simulink model "pendulum_ADRC_sim_sol"  (R2023b)
settings: Solver=ode3  StartTime=0.0  StopTime=20  FixedStep=0.01  RelTol=1e-3
values from neighbouring files (symbols this model uses):
  A = [ 0 1 ; 0 -a_m ]    [antenna_ADRC_par_sol.m]    (also in antenna_OFB_par_sol.m; pendulum_ADRC_par_sol.m = [ 0 , 1 , 0 ; 0 , 0 , 1 ; 0 , 0 , 0 ])
  a = [ m ; g ; l ; d ]    [pendulum_ADRC_par_sol.m]
  B = [ 0 ; Kl*Kg ]    [antenna_ADRC_par_sol.m]    (also in antenna_OFB_par_sol.m; pendulum_ADRC_par_sol.m = [ 0; b0 ; 0 ])
  b0 = 1/m    (= 0.02)    [pendulum_ADRC_par_sol.m]
  C = [ 1 , 0 ]    [antenna_ADRC_par_sol.m]    (also in antenna_OFB_par_sol.m; pendulum_ADRC_par_sol.m = [ 1 , 0 , 0 ])
  KD = 2*pole_CL    (= 3)    [pendulum_ADRC_par_sol.m]
  KP = pole_CL^2    (= 2.25)    [pendulum_ADRC_par_sol.m]
  L = acker(A',C',p_obs)'    [antenna_OFB_par_sol.m]    (also in pendulum_ADRC_par_sol.m = acker(A',C',poles_ESO)')
libraries: simulink_extras x3
settings Model: Creator=jerome  LastModifiedBy=jerome
settings ModelReferenceCC: EnableRefExpFcnMdlSchedulingChecks=on

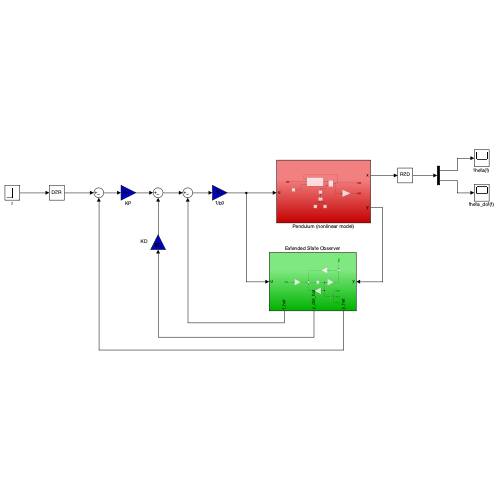
[thumbnail: Simulink's stored preview of the top-level diagram]
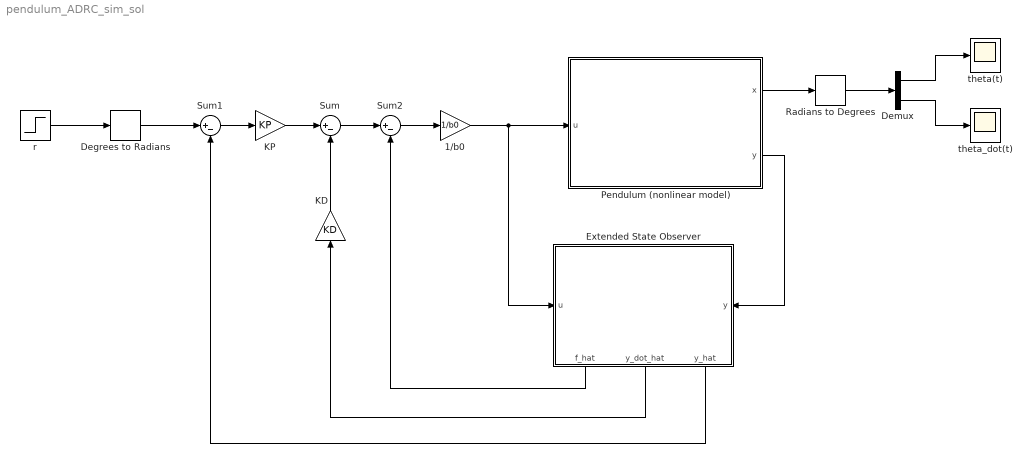
== system pendulum_ADRC_sim_sol ==
  1/b0 : Gain  Gain=1/b0
  Degrees to Radians : simulink_extras/Transformations/Degrees to Radians
  Demux : Demux  Outputs=2
  Extended State Observer : Subsystem
      settings: PortSchema="{\"entries\":[{\"content\":{\"sides\":[{\"content\":{\"connectorIds\":[\"In1\"]},\"type\":\"ConnectorPlacement.EquallySpacedRectSide\",\"uuid\":\"e39c489f-7ce3-4515-bfb3-5978cf16689b\"},{\"content\":{\"connectorIds\":[\"In2\"],\"side\":\"RIGHT\"},\"type\":\"ConnectorPlacement.EquallySpacedRectSide\",\"uuid\":\"c323375b-3042-4327-9d10-0e78d49b9c28\"},{\"content\":{\"connectorIds\":[],\"side\":\"TOP\"},\"type\":\"ConnectorPlacement.EquallySpacedRectSide\",\"uuid\":\"bc6e3c93-589b-408b-8e2a-2332a4933e23\"},{\"content\":{\"connectorIds\":[\"Out1\",\"Out2\",\"Out3\"],\"side\":\"BOTTOM\"},\"type\":\"ConnectorPlacement.EquallySpacedRectSide\",\"uuid\":\"0fa3e6d2-737b-4634-8e4c-4849dc2892cb\"}]},\"type\":\"ConnectorPlacement.EquallySpacedConnector\",\"uuid\":\"052b3b38-b01c-47b0-92b2-1f2c82c768d4\"}],\"packageUris\":[\"http://schema.mathworks.com/mf0/Connector/R2020b\"],\"version\":\"1.0\"}"
  KD : Gain  Gain=KD
  KP : Gain  Gain=KP
  Pendulum (nonlinear model) : Subsystem
  Radians to Degrees : simulink_extras/Transformations/Radians to Degrees
  Sum : Sum  Inputs=|+-
  Sum1 : Sum  Inputs=|+-
  Sum2 : Sum  Inputs=|+-
  r : Step  After=45  SampleTime=0
  theta(t) : Scope
  theta_dot(t) : Scope
  wires:
  KP/1 -> Sum/1
  Sum1/1 -> KP/1
  Extended State Observer/3(y_hat) -> Sum1/2
  Sum2/1 -> 1/b0/1
  Sum/1 -> Sum2/1
  Extended State Observer/1(f_hat) -> Sum2/2
  Extended State Observer/2(y_dot_hat) -> KD/1
  KD/1 -> Sum/2
  Pendulum (nonlinear model)/1(x) -> Radians to Degrees/1
  Radians to Degrees/1 -> Demux/1
  Demux/1 -> theta(t)/1
  Demux/2 -> theta_dot(t)/1
  Pendulum (nonlinear model)/2(y) -> Extended State Observer/2(y)
  1/b0/1 -> Extended State Observer/1(u), Pendulum (nonlinear model)/1(u)
  Degrees to Radians/1 -> Sum1/1
  r/1 -> Degrees to Radians/1

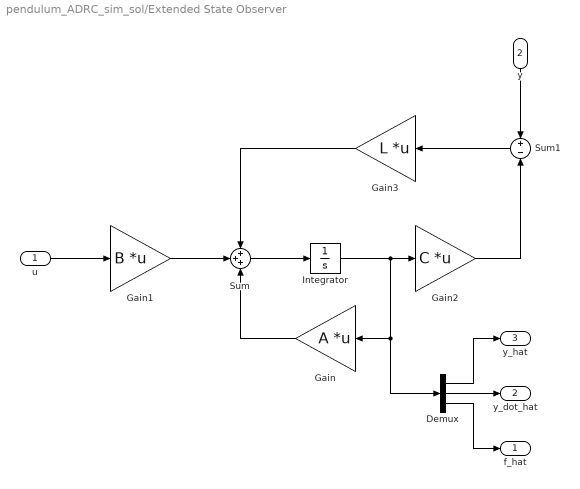
== system pendulum_ADRC_sim_sol/Extended State Observer ==
  u : Inport
  y : Inport  Port=2
  Demux : Demux  Outputs=3
  Gain : Gain  Gain=A  Multiplication=Matrix(K*u) (u vector)
  Gain1 : Gain  Gain=B  Multiplication=Matrix(K*u) (u vector)
  Gain2 : Gain  Gain=C  Multiplication=Matrix(K*u) (u vector)
  Gain3 : Gain  Gain=L  Multiplication=Matrix(K*u) (u vector)
  Integrator : Integrator  InitialCondition=zeros(3,1)
  Sum : Sum  Inputs=+++
  Sum1 : Sum  Inputs=+-
  f_hat : Outport
  y_dot_hat : Outport  Port=2
  y_hat : Outport  Port=3
  wires:
  Integrator/1 -> Gain2/1, Demux/1, Gain/1
  Demux/1 -> y_hat/1
  Sum/1 -> Integrator/1
  u/1 -> Gain1/1
  Gain/1 -> Sum/3
  Gain1/1 -> Sum/2
  Gain3/1 -> Sum/1
  Sum1/1 -> Gain3/1
  Gain2/1 -> Sum1/2
  y/1 -> Sum1/1
  Demux/3 -> f_hat/1
  Demux/2 -> y_dot_hat/1

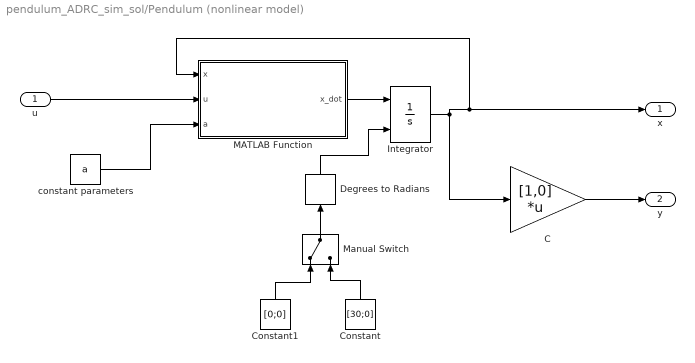
== system pendulum_ADRC_sim_sol/Pendulum (nonlinear model) ==
  u : Inport
  C : Gain  Gain=[1,0]  Multiplication=Matrix(K*u) (u vector)
  Constant : Constant  Value=[30;0]  VectorParams1D=off
  Constant1 : Constant  Value=[0;0]  VectorParams1D=off
  Degrees to Radians : simulink_extras/Transformations/Degrees to Radians
  Integrator : Integrator  InitialConditionSource=external  InitialCondition=[0.1;0]
  MATLAB Function : MATLAB Function  TreatAsAtomicUnit=on
  Manual Switch : ManualSwitch
  constant parameters : Constant  Value=a  VectorParams1D=off
  x : Outport
  y : Outport  Port=2
  wires:
  u/1 -> MATLAB Function/2(u)
  MATLAB Function/1(x_dot) -> Integrator/1
  Integrator/1 -> C/1, MATLAB Function/1(x), x/1
  constant parameters/1 -> MATLAB Function/3(a)
  C/1 -> y/1
  Constant/1 -> Manual Switch/2
  Degrees to Radians/1 -> Integrator/2
  Constant1/1 -> Manual Switch/1
  Manual Switch/1 -> Degrees to Radians/1

== matlab function pendulum_ADRC_sim_sol/Pendulum (nonlinear model)/MATLAB Function ==
  data: x input; u input; x_dot output; a input
function x_dot = f(x,u,a)

% a is the vector of constant parameters
m = a(1);
g = a(2);
l = a(3);
d = a(4);

x_dot = [ x(2) ; 1/(m*l^2)*(-m*g*l*sin(x(1))-d*x(2)+u) ];
